simulink model "RC_TOP"  (Simulink 9.2)
settings: Solver=ode1  StartTime=0.0  StopTime=5000000.0  FixedStep=0.1  RelTol=1e-3  EnableMultiTasking=on
settings Model: Creator=user  LastModifiedBy=user
settings DataIOCC: SignalLoggingSaveFormat=Dataset
settings DebuggingCC: UnderspecifiedInitializationDetection=Simplified  MergeDetectMultiDrivingBlocksExec=error  SolverPrmCheckMsg=warning  FcnCallInpInsideContextMsg=error  StateNameClashWarn=none
settings GRTTargetCC: CombineOutputUpdateFcns=on  GRTInterface=off
settings ConfigComp: CovSFcnEnable=off

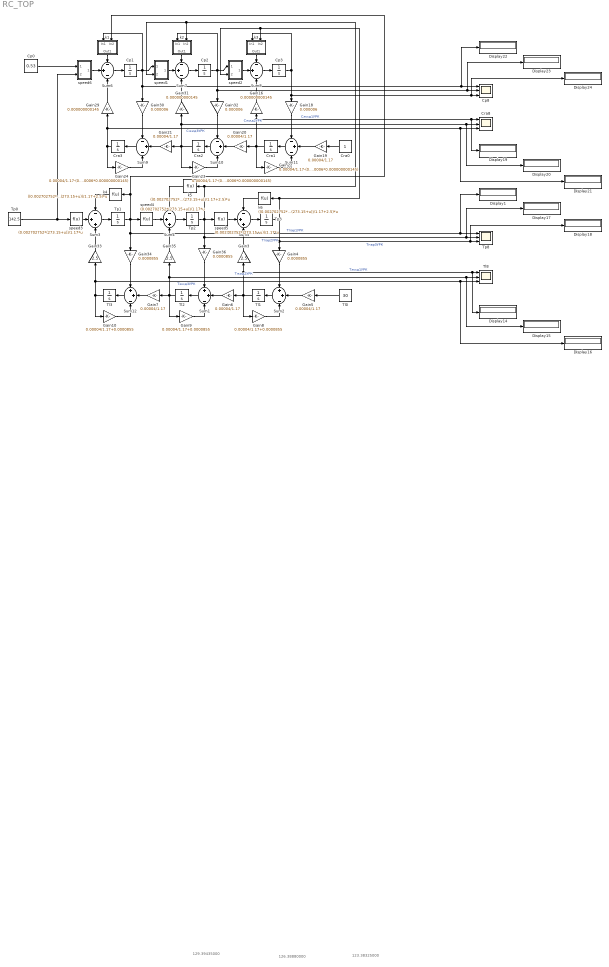
== system RC_TOP ==
  note: 129.39435000
  note: 126.38880000
  note: 123.38325000
  Cp0 : Constant  Value=0.53
  Cp1 : Integrator  InitialCondition=0.68200000
  Cp2 : Integrator  InitialCondition=0.83400000
  Cp3 : Integrator  InitialCondition=0.98600000
  Cp8 : Scope  NumInputPorts=3
  Cra0 : Constant
  Cra1 : Integrator  InitialCondition=0.88825000
  Cra2 : Integrator  InitialCondition=0.77650000
  Cra3 : Integrator  InitialCondition=0.66475000
  Cra8 : Scope  NumInputPorts=3
  Display{1,14..24} (12 alike) : Display
  Gain10 : Gain  Gain=0.00004/1.17+0.0000855
  Gain16 : Gain  Gain=0.000000000145
  Gain18 : Gain  Gain=0.000006
  Gain{5..7,19..21} (6 alike) : Gain  Gain=0.00004/1.17
  Gain22 : Gain  Gain=0.00004/1.17-(0.000006*0.000000000145)
  Gain23 : Gain  Gain=0.00004/1.17-(0.000006*0.000000000145)
  Gain24 : Gain  Gain=0.00004/1.17-(0.000006*0.000000000145)
  Gain29 : Gain  Gain=0.000000000145
  Gain3 : Gain  Gain=2.5
  Gain30 : Gain  Gain=0.000006
  Gain31 : Gain  Gain=0.000000000145
  Gain32 : Gain  Gain=0.000006
  Gain33 : Gain  Gain=2.5
  Gain34 : Gain  Gain=0.0000855
  Gain35 : Gain  Gain=2.5
  Gain36 : Gain  Gain=0.0000855
  Gain4 : Gain  Gain=0.0000855
  Gain8 : Gain  Gain=0.00004/1.17+0.0000855
  Gain9 : Gain  Gain=0.00004/1.17+0.0000855
  Sum1 : Sum  Inputs=++-
  Sum{6..11} (6 alike) : Sum  Inputs=-+-
  Sum12 : Sum  Inputs=++-
  Sum2 : Sum  Inputs=++-
  Sum3 : Sum  Inputs=-++
  Sum4 : Sum  Inputs=-++
  Sum5 : Sum  Inputs=-++
  Tl0 : Constant  Value=30
  Tl1 : Integrator  InitialCondition=57.25000000
  Tl2 : Integrator  InitialCondition=84.50000000
  Tl3 : Integrator  InitialCondition=111.75000000
  Tl8 : Scope  NumInputPorts=3
  Tp0 : Constant  Value=142.5
  Tp1 : Integrator  InitialCondition=118.20000000
  Tp2 : Integrator  InitialCondition=93.90000000
  Tp3 : Integrator  InitialCondition=69.60000000  IgnoreLimit=on
  Tp8 : Scope  NumInputPorts=3
  k1 : Subsystem
  k2 : Subsystem
  k3 : Subsystem
  k4 : Fcn  Expr=((0.002702752*(273.15+u))/1.17+2.5)*u
  k5 : Fcn  Expr=((0.002702752*(273.15+u))/1.17+2.5)*u
  k6 : Fcn  Expr=((0.002702752*(273.15+u))/1.17+2.5)*u
  speed1 : Subsystem
  speed2 : Subsystem
  speed3 : Fcn  Expr=(0.002702752*(273.15+u))/1.17*u
  speed4 : Fcn  Expr=(0.002702752*(273.15+u))/1.17*u
  speed5 : Fcn  Expr=(0.002702752*(273.15+u))/1.17*u
  speed6 : Subsystem
  wires:
  Sum6/1 -> Cp1/1
  speed1/1(Out1) -> Sum7/2
  Sum7/1 -> Cp2/1
  speed2/1(Out1) -> Sum8/2
  Sum8/1 -> Cp3/1
  Cp1/1 -> Cp8/1, Display22/1, Gain30/1, k1/1(In1), speed1/1(In1)
  Cp2/1 -> Display23/1, Cp8/2, Gain32/1, speed2/1(In1), k2/1(In1)
  Gain29/1 -> Sum6/3
  Cp3/1 -> Display24/1, Cp8/3, Gain18/1, k3/1(In1)
  Gain31/1 -> Sum7/3
  Gain16/1 -> Sum8/3
  Gain30/1 -> Sum9/1
  Gain32/1 -> Sum10/1
  Gain18/1 -> Sum11/1
  Gain19/1 -> Sum11/2
  Sum11/1 -> Cra1/1
  Cra1/1 -> Gain22/1, Gain20/1, Display19/1, Cra8/1, Gain16/1  "Cжид1УРК"
  Gain20/1 -> Sum10/2
  Sum10/1 -> Cra2/1
  Cra2/1 -> Gain23/1, Gain21/1, Display20/1, Cra8/2, Gain31/1  "Cжид2УРК"
  Gain21/1 -> Sum9/2
  Sum9/1 -> Cra3/1
  Cra3/1 -> Gain24/1, Display21/1, Cra8/3, Gain29/1  "Cжид3УРК"
  Gain22/1 -> Sum11/3
  Gain23/1 -> Sum10/3
  Gain24/1 -> Sum9/3
  speed3/1 -> Sum3/2
  k4/1 -> Sum3/1
  Sum3/1 -> Tp1/1
  speed4/1 -> Sum4/2
  k5/1 -> Sum4/1
  Sum4/1 -> Tp2/1
  speed5/1 -> Sum5/2
  k6/1 -> Sum5/1
  Sum5/1 -> Tp3/1
  Tp1/1 -> Display1/1, Tp8/1, Gain34/1, k4/1, k1/2(In2), speed4/1  "Tпар1УРК"
  Gain33/1 -> Sum3/3
  Tp3/1 -> Display18/1, Tp8/3, Gain4/1, k6/1, k3/2(In2), speed2/2(In2)  "Tпар3УРК"
  Gain35/1 -> Sum4/3
  Gain3/1 -> Sum5/3
  Gain34/1 -> Sum12/1
  Gain36/1 -> Sum1/1
  Gain4/1 -> Sum2/1
  Gain5/1 -> Sum2/2
  Sum2/1 -> Tl1/1
  Tl1/1 -> Gain8/1, Gain6/1, Display14/1, Tl8/1, Gain3/1  "Tжид1УРК"
  Gain6/1 -> Sum1/2
  Sum1/1 -> Tl2/1
  Tl2/1 -> Gain9/1, Gain7/1, Display15/1, Tl8/2, Gain35/1  "Tжид2УРК"
  Gain7/1 -> Sum12/2
  Sum12/1 -> Tl3/1
  Tl3/1 -> Gain10/1, Display16/1, Tl8/3, Gain33/1  "Tжид3УРК"
  Gain8/1 -> Sum2/3
  Gain9/1 -> Sum1/3
  Gain10/1 -> Sum12/3
  speed6/1(Out1) -> Sum6/2
  Cp0/1 -> speed6/1(In1)
  k1/1(Out1) -> Sum6/1
  k2/1(Out1) -> Sum7/1
  k3/1(Out1) -> Sum8/1
  Cra0/1 -> Gain19/1
  Tl0/1 -> Gain5/1
  Tp2/1 -> Display17/1, Tp8/2, Gain36/1, k5/1, k2/2(In2), speed1/2(In2), speed5/1  "Tпар2УРК"
  Tp0/1 -> speed6/2(In2), speed3/1

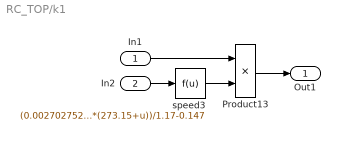
== system RC_TOP/k1 ==
  In1 : Inport
  In2 : Inport  Port=2
  Product13 : Product  SaturateOnIntegerOverflow=on  InputSameDT=on  OutDataTypeStr=Inherit: Same as first input
  speed3 : Fcn  Expr=(0.002702752*(273.15+u))/1.17-0.147
  Out1 : Outport
  wires:
  Product13/1 -> Out1/1
  speed3/1 -> Product13/2
  In2/1 -> speed3/1
  In1/1 -> Product13/1

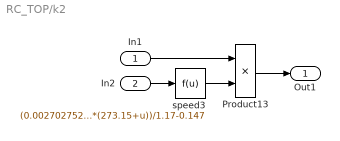
== system RC_TOP/k2 ==
  In1 : Inport
  In2 : Inport  Port=2
  Product13 : Product  SaturateOnIntegerOverflow=on  InputSameDT=on  OutDataTypeStr=Inherit: Same as first input
  speed3 : Fcn  Expr=(0.002702752*(273.15+u))/1.17-0.147
  Out1 : Outport
  wires:
  In1/1 -> Product13/1
  In2/1 -> speed3/1
  speed3/1 -> Product13/2
  Product13/1 -> Out1/1

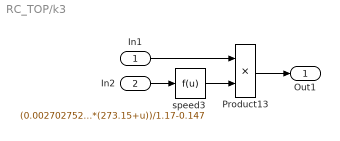
== system RC_TOP/k3 ==
  In1 : Inport
  In2 : Inport  Port=2
  Product13 : Product  SaturateOnIntegerOverflow=on  InputSameDT=on  OutDataTypeStr=Inherit: Same as first input
  speed3 : Fcn  Expr=(0.002702752*(273.15+u))/1.17-0.147
  Out1 : Outport
  wires:
  Product13/1 -> Out1/1
  speed3/1 -> Product13/2
  In2/1 -> speed3/1
  In1/1 -> Product13/1

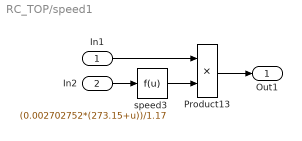
== system RC_TOP/speed1 ==
  In1 : Inport
  In2 : Inport  Port=2
  Product13 : Product  SaturateOnIntegerOverflow=on  InputSameDT=on  OutDataTypeStr=Inherit: Same as first input
  speed3 : Fcn  Expr=(0.002702752*(273.15+u))/1.17
  Out1 : Outport
  wires:
  Product13/1 -> Out1/1
  speed3/1 -> Product13/2
  In2/1 -> speed3/1
  In1/1 -> Product13/1

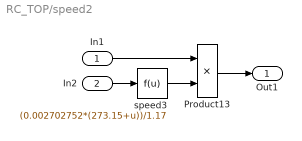
== system RC_TOP/speed2 ==
  In1 : Inport
  In2 : Inport  Port=2
  Product13 : Product  SaturateOnIntegerOverflow=on  InputSameDT=on  OutDataTypeStr=Inherit: Same as first input
  speed3 : Fcn  Expr=(0.002702752*(273.15+u))/1.17
  Out1 : Outport
  wires:
  In1/1 -> Product13/1
  In2/1 -> speed3/1
  speed3/1 -> Product13/2
  Product13/1 -> Out1/1

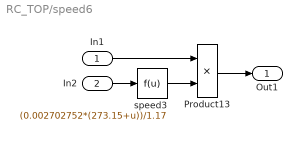
== system RC_TOP/speed6 ==
  In1 : Inport
  In2 : Inport  Port=2
  Product13 : Product  SaturateOnIntegerOverflow=on  InputSameDT=on  OutDataTypeStr=Inherit: Same as first input
  speed3 : Fcn  Expr=(0.002702752*(273.15+u))/1.17
  Out1 : Outport
  wires:
  In1/1 -> Product13/1
  In2/1 -> speed3/1
  speed3/1 -> Product13/2
  Product13/1 -> Out1/1
